simulink library "CTRL_LO_ST1_LGTFDIS"  (R2023b)
settings: Solver=VariableStepAuto  StartTime=0.0  StopTime=10.0  RelTol=1e-3
settings Model: Creator=blatak  LastModifiedBy=blatak

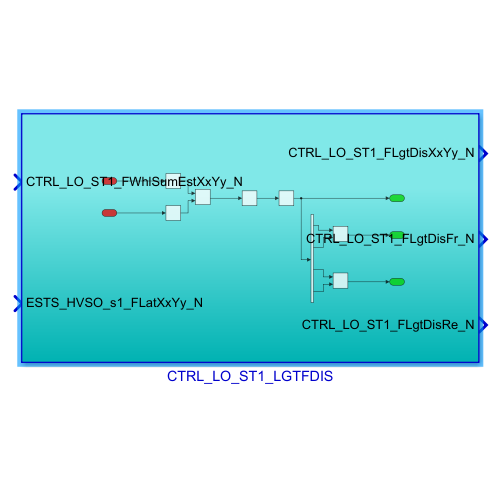
[thumbnail: Simulink's stored preview of the top-level diagram]
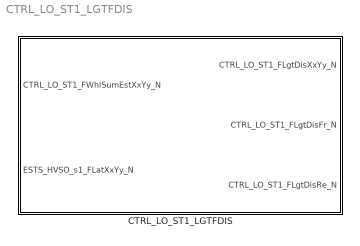
== system CTRL_LO_ST1_LGTFDIS ==
  CTRL_LO_ST1_LGTFDIS : Subsystem

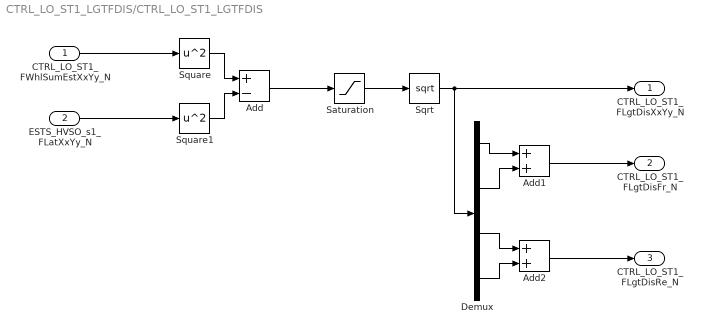
== system CTRL_LO_ST1_LGTFDIS/CTRL_LO_ST1_LGTFDIS ==
  CTRL_LO_ST1_FWhlSumEstXxYy_N : Inport
  ESTS_HVSO_s1_FLatXxYy_N : Inport  Port=2
  Add : Sum  Inputs=+-
  Add1 : Sum
  Add2 : Sum
  Demux : Demux
  Saturation : Saturate  UpperLimit=inf  LowerLimit=0
  Sqrt : Sqrt
  Square : Math  Operator=square
  Square1 : Math  Operator=square
  CTRL_LO_ST1_FLgtDisXxYy_N : Outport
  CTRL_LO_ST1_FLgtDisFr_N : Outport  Port=2
  CTRL_LO_ST1_FLgtDisRe_N : Outport  Port=3
  wires:
  Square1/1 -> Add/2
  Square/1 -> Add/1
  CTRL_LO_ST1_FWhlSumEstXxYy_N/1 -> Square/1
  ESTS_HVSO_s1_FLatXxYy_N/1 -> Square1/1
  Sqrt/1 -> Demux/1, CTRL_LO_ST1_FLgtDisXxYy_N/1
  Add/1 -> Saturation/1
  Saturation/1 -> Sqrt/1
  Demux/3 -> Add2/1
  Demux/4 -> Add2/2
  Demux/2 -> Add1/2
  Demux/1 -> Add1/1
  Add1/1 -> CTRL_LO_ST1_FLgtDisFr_N/1
  Add2/1 -> CTRL_LO_ST1_FLgtDisRe_N/1
